simulink model "modelo_verificado"  (R2023b)
settings: Solver=VariableStepAuto  StartTime=0.0  StopTime=10.0  RelTol=1e-3
undefined symbols (not defined in the file): alpha, beta, gamma, I0, R0, rho, S0

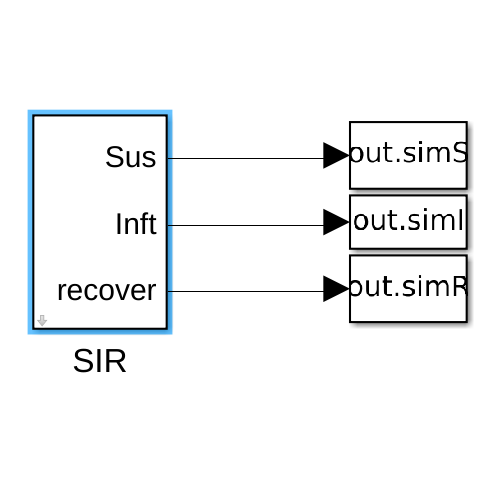
[thumbnail: Simulink's stored preview of the top-level diagram]
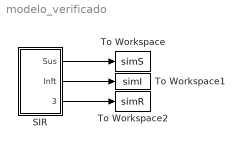
== system modelo_verificado ==
  SIR : Subsystem  mask(Parámetros){S0=S0, I0=I0, R0=R0, alpha=alpha, beta=beta, rho=rho, gamma=gamma}
      mask prompts: S0 "S(0)"; I0 "I(0)"; R0 "R(0)"; alpha "alpha(α)"; beta "beta(β)"; rho "rho(ρ)"; gamma "gamma(ɣ)"
      mask help:
      | Variables
      | Condiciones iniciales:
      | S(0), I(0) y R(0), donde:
      | 1. S - Los susceptibles de enterarse del chisme
      | 2. I - Los infectados (chismosos)
      | 3. R - Recuperados de la infección (ya no creen en el chisme)
      | β : la razón a la que se difunde el rumor
      | 1-ρ : el porcentaje de la población que desestiman el (rumor con solo oírlo)
      | γ : a razón a la que los infectados desestiman el rumor
      | α : la razón de persuasión de los Infectados(sobre los recupe
      mask Help:
      | <p style="color: black;">&beta;: la tasa a la que se difunde el rumor</p>
      | <p style="color: black;">(1-&rho;): el porcentaje de la población que desestima el rumor con solo oírlo</p>
      | <p style="color: black;">&gamma;: la tasa a la que los infectados desestiman el rumor</p>
      | <p style="color: black;">&alpha;: la tasa de persuasión de los infectados sobre los recuperados</p>
  To Workspace : ToWorkspace  VariableName=simS  SaveFormat=Timeseries  SampleTime=-1
  To Workspace1 : ToWorkspace  VariableName=simI  SaveFormat=Timeseries  SampleTime=-1
  To Workspace2 : ToWorkspace  VariableName=simR  SaveFormat=Timeseries  SampleTime=-1
  wires:
  SIR/3(recover) -> To Workspace2/1
  SIR/2(Inft) -> To Workspace1/1
  SIR/1(Sus) -> To Workspace/1

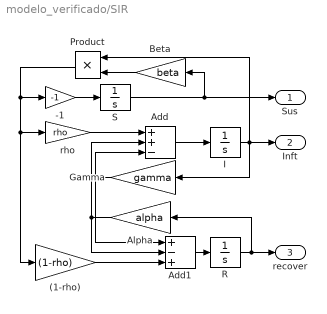
== system modelo_verificado/SIR ==
  (1-rho) : Gain  Gain=(1-rho)
  -1 : Gain  Gain=-1
  Add : Sum  Inputs=++-
  Add1 : Sum  Inputs=+-+
  Alpha : Gain  Gain=alpha
  Beta : Gain  Gain=beta
  Gamma : Gain  Gain=gamma
  I : Integrator  InitialCondition=I0
  Product : Product
  R : Integrator  InitialCondition=R0
  S : Integrator  InitialCondition=S0
  rho : Gain  Gain=rho
  Sus : Outport
  Inft : Outport  Port=2
  recover : Outport  Port=3
  wires:
  Product/1 -> (1-rho)/1, rho/1, -1/1
  S/1 -> Beta/1, Sus/1
  Add/1 -> I/1
  R/1 -> recover/1, Alpha/1
  (1-rho)/1 -> Add1/3
  Beta/1 -> Product/2
  rho/1 -> Add/1
  -1/1 -> S/1
  Add1/1 -> R/1
  Alpha/1 -> Add1/2, Add/2
  Gamma/1 -> Add1/1, Add/3
  I/1 -> Product/1, Inft/1, Gamma/1
